simulink model "Final_ShipModel_R19"  (R2019a)
settings: Solver=VariableStepAuto  StartTime=0.0  StopTime=100  RelTol=1e-3
libraries: simulink x3, mssSimulink x2
settings Model: PacingRate=10  Creator=Lenovo  LastModifiedBy=LENOVO
settings DebuggingCC: UnconnectedInputMsg=none  UnconnectedOutputMsg=none  UnconnectedLineMsg=none  SFMachineParentedDataDiag=error

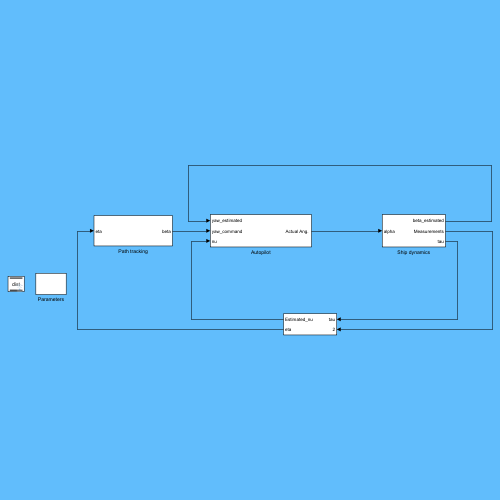
[thumbnail: Simulink's stored preview of the top-level diagram]
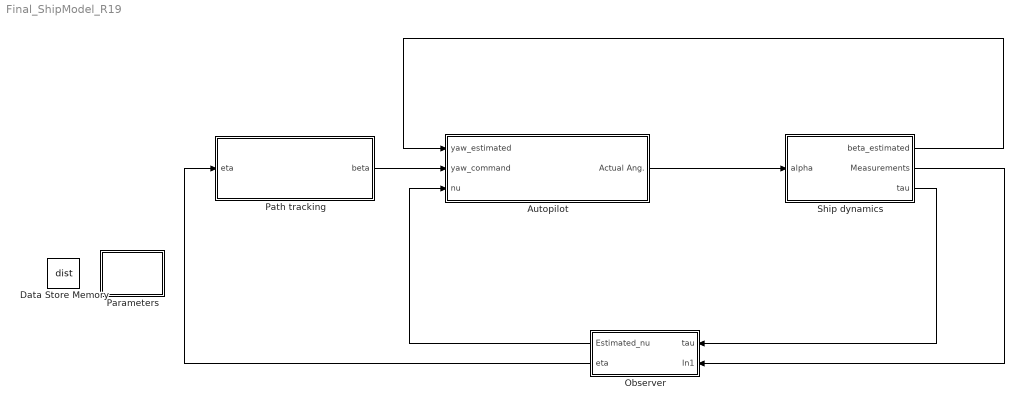
== system Final_ShipModel_R19 ==
  Autopilot : Subsystem
  Data Store Memory : DataStoreMemory  DataStoreName=dist  WriteAfterWriteMsg=warning  InitialValue=1000  ShowAdditionalParam=off  OutDataTypeStr=double
  Observer : Subsystem
  Parameters : Subsystem
  Path tracking : Subsystem
  Ship dynamics : Subsystem
  wires:
  Path tracking/1(beta) -> Autopilot/2(yaw_command)
  Autopilot/1("Actual Ang. ") -> Ship dynamics/1(alpha)
  Ship dynamics/1(beta_estimated) -> Autopilot/1(yaw_estimated)
  Ship dynamics/2(Measurements) -> Observer/2(In1)
  Ship dynamics/3(tau) -> Observer/1(tau)
  Observer/2(eta) -> Path tracking/1(eta)
  Observer/1(Estimated_nu) -> Autopilot/3(nu)

== system Final_ShipModel_R19/Autopilot ==
  yaw_estimated : Inport
  yaw_command : Inport  Port=2
  nu : Inport  Port=3
  Autopilot : Subsystem
  Constant3 : Constant  Value=0
  Fin/Rudder Machinery : Subsystem  AncestorBlock=mssSimulink/Modelling/Control Surfaces/Fin//Rudder Machinery  mask(Rudder Machinery){Dmax=20, Dvmax=2*pi*1000/180, tc=.1}
      mask prompts: Dmax "Max. Rudder Angle (rad):"; Dvmax "Max. Rudder Rate (rad/sec.):"; tc "Time constant (sec):"
      mask help:
      | Model of van Amerongen for rudder machiery
      | Copyright (C) 2005 NTNU
      | Author: Tristan Perez
      mask Help: Rudder machinery model of Van Amerongen accounting for saturation and rate limit.
  Selector : Selector  InputPortWidth=3  IndexOptions=Index vector (dialog)  Indices=[3]  OutputSizes=1
  "Actual Ang. " : Outport
  wires:
  Selector/1 -> Autopilot/4(r_estimated)  "r"
  Constant3/1 -> Autopilot/3(r_command)
  yaw_estimated/1 -> Autopilot/2(yaw_estimated)
  Fin/Rudder Machinery/1("Actual Ang. ") -> "Actual Ang. "/1
  Autopilot/1(rudder_angle_command) -> Fin/Rudder Machinery/1(Angle Comm)
  nu/1 -> Selector/1
  yaw_command/1 -> Autopilot/1(yaw_command)

== system Final_ShipModel_R19/Observer ==
  tau : Inport
  In1 : Inport  Port=2
  Kalman gain : Gain  Gain=-10
  Sensor Model(Supply vessel2) : Subsystem  AncestorBlock=mssSimulink/Marine craft models/Supply vessel
  Sum : Sum  Inputs=-+|
  Estimated_nu : Outport
  eta : Outport  Port=2
  wires:
  Kalman gain/1 -> Sensor Model(Supply vessel2)/2(Error*Kalman Gain)
  Sensor Model(Supply vessel2)/1(Estimated_eta) -> Sum/2, eta/1  "eta"
  In1/1 -> Sum/1
  Sensor Model(Supply vessel2)/2(Estimated_nu) -> Estimated_nu/1
  tau/1 -> Sensor Model(Supply vessel2)/1(tau)
  Sum/1 -> Kalman gain/1

== system Final_ShipModel_R19/Parameters ==
  Izz : Constant  Value=47.934*10^6
  Izz1 : Constant  Value=47.934*10^6*0.8
  Mass : Constant  Value=357.0*1014
  Mass1 : Constant  Value=357.0*1014*0.8
  tag scope: Izz1=global, Izz=global, Mass1=global, Mass=global
  wires:
  Mass/1 -> [Mass]
  Izz/1 -> [Izz]
  Izz1/1 -> [Izz1]
  Mass1/1 -> [Mass1]

== system Final_ShipModel_R19/Path tracking ==
  eta : Inport
  Data Store Read : DataStoreRead  DataStoreName=dist
  Path assigning : MATLAB Function  TreatAsAtomicUnit=on
  Path following : Subsystem
  Path generation : Constant  Value=[500 0; 500 2000; 1000 1500; 2000 0]
  Stop Simulation1 : Stop
  beta : Outport
  wires:
  Path generation/1 -> Path assigning/1(path)
  Data Store Read/1 -> Path assigning/2(dist)
  Path assigning/1(wp1) -> Path following/2(Waypoint 1)
  Path assigning/3(stop) -> Stop Simulation1/1
  Path assigning/2(wp2) -> Path following/3(Waypoint 2)
  eta/1 -> Path following/1(Ship Position)
  Path following/1(beta) -> beta/1

== system Final_ShipModel_R19/Ship dynamics ==
  alpha : Inport
  Noises : Subsystem
  Pod-Propellers : Subsystem
  Supply vessel dynamics : Subsystem
  beta_estimated : Outport
  Measurements : Outport  Port=2
  tau : Outport  Port=3
  wires:
  Pod-Propellers/1(tau) -> Supply vessel dynamics/1(tau), tau/1
  Supply vessel dynamics/3(nu) -> Pod-Propellers/2(nu1)
  Supply vessel dynamics/2(beta_estimated) -> beta_estimated/1
  Noises/1(Noises) -> Measurements/1
  Supply vessel dynamics/1(eta) -> Noises/1(Signal)
  alpha/1 -> Pod-Propellers/1(alpha)

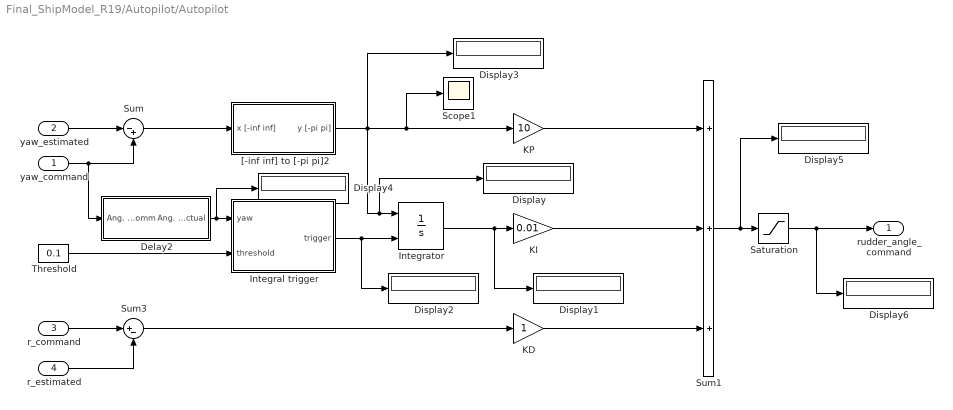
== system Final_ShipModel_R19/Autopilot/Autopilot ==
  yaw_command : Inport
  yaw_estimated : Inport  Port=2
  r_command : Inport  Port=3
  r_estimated : Inport  Port=4
  Delay2 : Subsystem
  Display{,1..6} (7 alike) : Display
  Integral trigger : MATLAB Function  TreatAsAtomicUnit=on
  Integrator : Integrator  ExternalReset=level hold  LimitOutput=on  UpperSaturationLimit=deg2rad(20)  LowerSaturationLimit=deg2rad(-20)
  KD : Gain
  KI : Gain  Gain=0.01
  KP : Gain  Gain=10
  Saturation : Saturate  UpperLimit=deg2rad(20)  LowerLimit=deg2rad(-20)
  Scope1 : Scope
  Sum : Sum  Inputs=|-+
  Sum1 : Sum  Inputs=+++  InputSameDT=on  SaturateOnIntegerOverflow=on  OutDataTypeStr=Inherit: Same as first input
  Sum3 : Sum  Inputs=|+-  InputSameDT=on  SaturateOnIntegerOverflow=on  OutDataTypeStr=Inherit: Same as first input
  Threshold : Constant  Value=0.1
  "[-inf inf] to [-pi pi]2" : Subsystem  AncestorBlock=mssSimulink/Utilities/Math Operations/[-inf inf] to [-pi pi]  mask([-inf inf] to [-pi pi]){}
      mask help: Converts an angle in rad to (-pi pi)
  rudder_angle_command : Outport
  wires:
  Integrator/1 -> Display1/1, KI/1
  KD/1 -> Sum1/3
  Sum/1 -> "[-inf inf] to [-pi pi]2"/1(x [-inf inf])
  Sum3/1 -> KD/1
  "[-inf inf] to [-pi pi]2"/1(y [-pi pi]) -> Scope1/1, KP/1, Display3/1, Display/1, Integrator/1
  KI/1 -> Sum1/2
  Sum1/1 -> Display5/1, Saturation/1
  r_estimated/1 -> Sum3/2
  r_command/1 -> Sum3/1
  yaw_estimated/1 -> Sum/1
  KP/1 -> Sum1/1
  Integral trigger/1(trigger) -> Display2/1, Integrator/2
  Threshold/1 -> Integral trigger/2(threshold)
  yaw_command/1 -> Sum/2, Delay2/1(Ang. Comm)
  Delay2/1(Ang. Actual) -> Display4/1, Integral trigger/1(yaw)
  Saturation/1 -> Display6/1, rudder_angle_command/1

== system Final_ShipModel_R19/Autopilot/Fin//Rudder Machinery ==
  Angle Comm : Inport
  Gain : Gain  Gain=1/tc  SaturateOnIntegerOverflow=on  OutDataTypeStr=Inherit: Same as input  ParamDataTypeStr=Inherit: Same as input
  Gain1 : Gain  Gain=-1
  Integrator : Integrator
  Saturation : Saturate  UpperLimit=deg2rad(30)  LowerLimit=-deg2rad(30)
  Saturation1 : Saturate  UpperLimit=deg2rad(Dmax)  LowerLimit=deg2rad(-Dmax)
  Sum : Sum  Inputs=|+-  InputSameDT=on  SaturateOnIntegerOverflow=on  OutDataTypeStr=Inherit: Same as first input
  "Actual Ang. " : Outport  VectorParamsAs1DForOutWhenUnconnected=off
  wires:
  Gain/1 -> Saturation/1
  Sum/1 -> Gain/1
  Integrator/1 -> Sum/2, Gain1/1
  Saturation1/1 -> Sum/1
  Saturation/1 -> Integrator/1
  Angle Comm/1 -> Saturation1/1
  Gain1/1 -> "Actual Ang. "/1

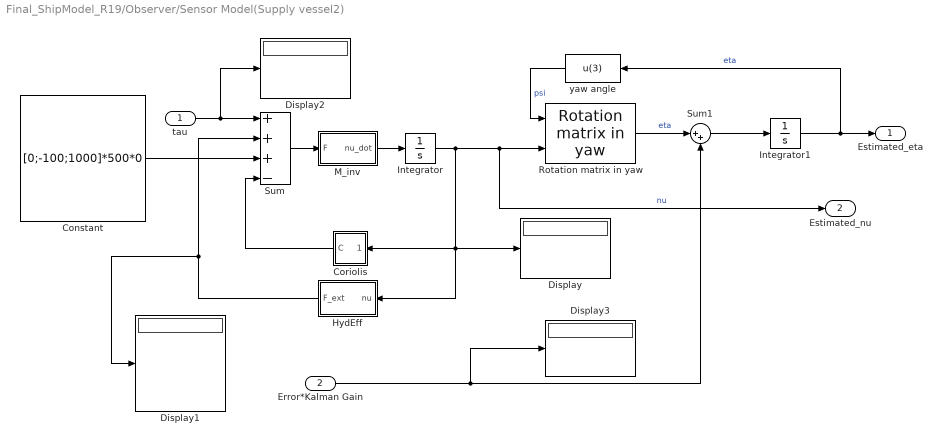
== system Final_ShipModel_R19/Observer/Sensor Model(Supply vessel2) ==
  tau : Inport
  Error*Kalman Gain : Inport  Port=2
  Constant : Constant  Value=[0;-100;1000]*500*0
  Coriolis : Subsystem
  Display{,1..3} (4 alike) : Display
  HydEff : Subsystem
  Integrator : Integrator  InitialCondition=[0 1 0]
  Integrator1 : Integrator
  M_inv : Subsystem
  "Rotation matrix in yaw " : mssSimulink/Modelling/Kinematics/Rotation matrix in yaw 
  Sum : Sum  Inputs=+++-  InputSameDT=on  SaturateOnIntegerOverflow=on  OutDataTypeStr=Inherit: Same as first input
  Sum1 : Sum  Inputs=|++
  yaw angle : Fcn  Expr=u(3)
  Estimated_eta : Outport  InitialOutput=0  VectorParamsAs1DForOutWhenUnconnected=off
  Estimated_nu : Outport  Port=2  InitialOutput=0  VectorParamsAs1DForOutWhenUnconnected=off
  wires:
  Sum/1 -> M_inv/1(F)
  M_inv/1(nu_dot) -> Integrator/1
  tau/1 -> Display2/1, Sum/1
  yaw angle/1 -> "Rotation matrix in yaw "/1  "psi"
  Integrator/1 -> Estimated_nu/1, "Rotation matrix in yaw "/2, Display/1, HydEff/1(nu), Coriolis/1(nu)  "nu"
  HydEff/1(F_ext) -> Display1/1, Sum/2
  Coriolis/1(C) -> Sum/4
  Constant/1 -> Sum/3
  Integrator1/1 -> Estimated_eta/1, yaw angle/1  "eta"
  Error*Kalman Gain/1 -> Display3/1, Sum1/2
  Sum1/1 -> Integrator1/1
  "Rotation matrix in yaw "/1 -> Sum1/1  "eta"

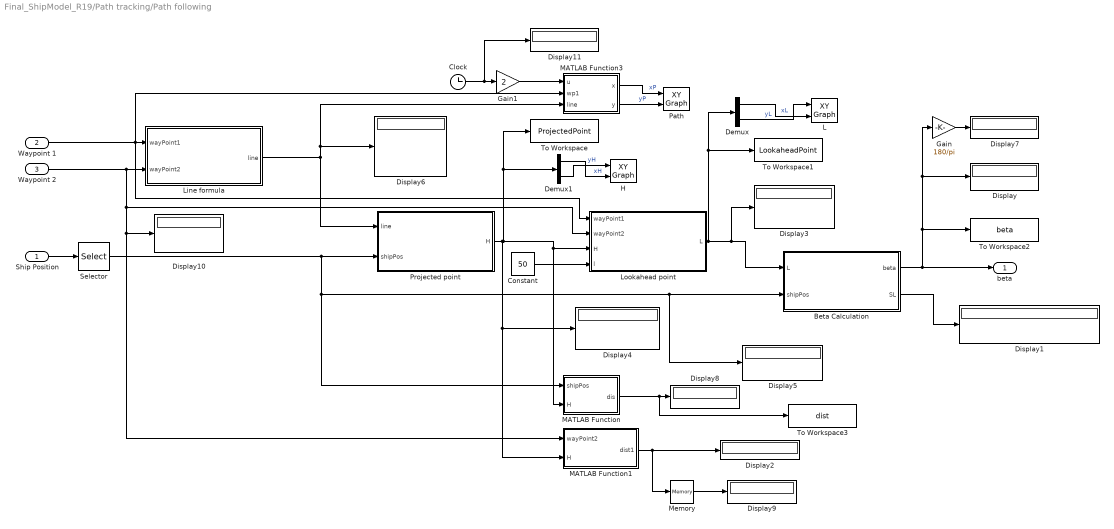
== system Final_ShipModel_R19/Path tracking/Path following ==
  Ship Position : Inport
  Waypoint 1 : Inport  Port=2
  Waypoint 2 : Inport  Port=3
  Beta Calculation : MATLAB Function  TreatAsAtomicUnit=on
  Clock : Clock
  Constant : Constant  Value=50
  Demux : Demux  Outputs=2
  Demux1 : Demux  Outputs=2
  Display{,1..11} (12 alike) : Display
  Gain : Gain  Gain=180/pi
  Gain1 : Gain  Gain=2
  H : simulink/Sinks/XY Graph  xmin=-1  xmax=1  ymin=-1  ymax=1  st=-1
  L : simulink/Sinks/XY Graph  xmin=-1  xmax=1  ymin=-1  ymax=1  st=-1
  Line formula : MATLAB Function  TreatAsAtomicUnit=on
  Lookahead point : MATLAB Function  TreatAsAtomicUnit=on
  MATLAB Function : MATLAB Function  TreatAsAtomicUnit=on
  MATLAB Function1 : MATLAB Function  TreatAsAtomicUnit=on
  MATLAB Function3 : MATLAB Function  TreatAsAtomicUnit=on
  Memory : Memory
  Path : simulink/Sinks/XY Graph  xmin=-1  xmax=1  ymin=-1  ymax=1  st=-1
  Projected point : MATLAB Function  TreatAsAtomicUnit=on
  Selector : Selector  InputPortWidth=3  IndexOptions=Index vector (dialog)  Indices=[1 2]  OutputSizes=1
  To Workspace : ToWorkspace  VariableName=ProjectedPoint  SaveFormat=Timeseries  SampleTime=-1
  To Workspace1 : ToWorkspace  VariableName=LookaheadPoint  SaveFormat=Timeseries  SampleTime=-1
  To Workspace2 : ToWorkspace  VariableName=beta  SaveFormat=Timeseries  SampleTime=-1
  To Workspace3 : ToWorkspace  VariableName=dist  SaveFormat=Timeseries  SampleTime=-1
  beta : Outport
  wires:
  Waypoint 1/1 -> Lookahead point/1(wayPoint1), Line formula/1(wayPoint1), MATLAB Function3/2(wp1)
  Waypoint 2/1 -> MATLAB Function1/1(wayPoint2), Display10/1, Lookahead point/2(wayPoint2), Line formula/2(wayPoint2)
  Ship Position/1 -> Selector/1
  Projected point/1(H) -> Display4/1, MATLAB Function1/2(H), To Workspace/1, Demux1/1, MATLAB Function/2(H), Lookahead point/3(H)
  Constant/1 -> Lookahead point/4(l)
  Lookahead point/1(L) -> To Workspace1/1, Demux/1, Display3/1, Beta Calculation/1(L)
  Beta Calculation/1(beta) -> beta/1, To Workspace2/1, Display/1, Gain/1
  Beta Calculation/2(SL) -> Display1/1
  Selector/1 -> Display5/1, Beta Calculation/2(shipPos), MATLAB Function/1(shipPos), Projected point/2(shipPos)
  Gain/1 -> Display7/1
  Gain1/1 -> MATLAB Function3/1(u)
  Clock/1 -> Display11/1, Gain1/1
  Line formula/1(line) -> Projected point/1(line), MATLAB Function3/3(line), Display6/1
  MATLAB Function3/2(y) -> Path/2  "yP"
  Demux/1 -> L/2  "xL"
  Demux/2 -> L/1  "yL"
  Demux1/1 -> H/2  "xH"
  Demux1/2 -> H/1  "yH"
  MATLAB Function/1(dis) -> To Workspace3/1, Display8/1
  MATLAB Function3/1(x) -> Path/1  "xP"
  MATLAB Function1/1(dist1) -> Display2/1, Memory/1
  Memory/1 -> Display9/1

== system Final_ShipModel_R19/Ship dynamics/Noises ==
  Signal : Inport
  Amplitude : Constant  Value=0
  Clock : Clock
  Mux1 : Mux  Inputs=3
  Sine Wave : Sin  TimeSource=Use external signal  Frequency=2  SampleTime=0
  Sum1 : Sum  Inputs=|++
  Noises : Outport
  wires:
  Signal/1 -> Sum1/1
  Clock/1 -> Sine Wave/1
  Sine Wave/1 -> Mux1/1, Mux1/2
  Sum1/1 -> Noises/1
  Mux1/1 -> Sum1/2
  Amplitude/1 -> Mux1/3

== system Final_ShipModel_R19/Ship dynamics/Pod-Propellers ==
  alpha : Inport
  nu1 : Inport  Port=2
  Add : Sum
  Propeller speed : Constant  Value=200
  propL : Subsystem
  propR : Subsystem
  tau : Outport
  wires:
  nu1/1 -> propL/1(nu), propR/1(nu1)
  alpha/1 -> propR/2(alpha1), propL/2(alpha)
  Propeller speed/1 -> propL/3(RPM), propR/3(RPM1)
  Add/1 -> tau/1
  propL/1(tau) -> Add/2
  propR/1(tau1) -> Add/1

== system Final_ShipModel_R19/Ship dynamics/Supply vessel dynamics ==
  tau : Inport
  MATLAB Function : MATLAB Function  TreatAsAtomicUnit=on
  Supply vessel : Subsystem  AncestorBlock=mssSimulink/Marine craft models/Supply vessel
  eta : Outport
  beta_estimated : Outport  Port=2
  nu : Outport  Port=3
  wires:
  MATLAB Function/1(beta_estimated) -> beta_estimated/1
  Supply vessel/3(velo) -> MATLAB Function/1(velo)
  tau/1 -> Supply vessel/1(tau)
  Supply vessel/1(eta) -> eta/1  "eta"
  Supply vessel/2(nu) -> nu/1

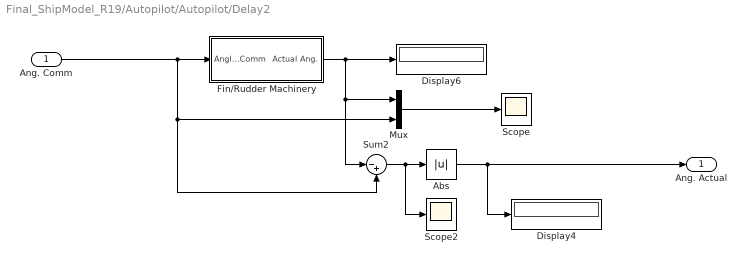
== system Final_ShipModel_R19/Autopilot/Autopilot/Delay2 ==
  Ang. Comm : Inport
  Abs : Abs  ZeroCross=off
  Display4 : Display
  Display6 : Display
  Fin/Rudder Machinery : Subsystem  AncestorBlock=mssSimulink/Modelling/Control Surfaces/Fin//Rudder Machinery  mask(Rudder Machinery){Dmax=20, Dvmax=0.05, tc=.005}
      mask prompts: Dmax "Max. Rudder Angle (rad):"; Dvmax "Max. Rudder Rate (rad/sec.):"; tc "Time constant (sec):"
      mask help:
      | Model of van Amerongen for rudder machiery
      | Copyright (C) 2005 NTNU
      | Author: Tristan Perez
      mask Help: Rudder machinery model of Van Amerongen accounting for saturation and rate limit.
  Mux : Mux  Inputs=2
  Scope : Scope
  Scope2 : Scope
  Sum2 : Sum  Inputs=|-+
  Ang. Actual : Outport
  wires:
  Sum2/1 -> Scope2/1, Abs/1
  Ang. Comm/1 -> Fin/Rudder Machinery/1(Angle Comm), Sum2/2, Mux/2
  Fin/Rudder Machinery/1("Actual Ang. ") -> Sum2/1, Mux/1, Display6/1
  Abs/1 -> Ang. Actual/1, Display4/1
  Mux/1 -> Scope/1

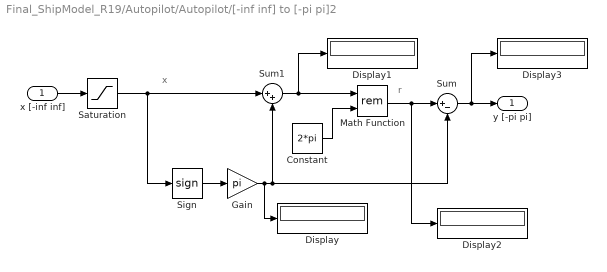
== system Final_ShipModel_R19/Autopilot/Autopilot/[-inf inf] to [-pi pi]2 ==
  note: x
  note: r
  x [-inf inf] : Inport
  Constant : Constant  Value=2*pi
  Display{,1..3} (4 alike) : Display
  Gain : Gain  Gain=pi  SaturateOnIntegerOverflow=on  OutDataTypeStr=Inherit: Same as input  ParamDataTypeStr=Inherit: Same as input
  Math Function : Math  Operator=rem  SaturateOnIntegerOverflow=on
  Saturation : Saturate  UpperLimit=1e10  LowerLimit=-1e10
  Sign : Signum
  Sum : Sum  Inputs=|+-  SaturateOnIntegerOverflow=on
  Sum1 : Sum  Inputs=|++  SaturateOnIntegerOverflow=on
  y [-pi pi] : Outport  VectorParamsAs1DForOutWhenUnconnected=off
  wires:
  x [-inf inf]/1 -> Saturation/1
  Sign/1 -> Gain/1
  Gain/1 -> Display/1, Sum/2, Sum1/2
  Sum1/1 -> Display1/1, Math Function/1
  Constant/1 -> Math Function/2
  Sum/1 -> Display3/1, y [-pi pi]/1
  Saturation/1 -> Sum1/1, Sign/1
  Math Function/1 -> Display2/1, Sum/1

== system Final_ShipModel_R19/Observer/Sensor Model(Supply vessel2)/Coriolis ==
  nu : Inport
  Demux : Demux  Outputs=3
  Display : Display
  MATLAB Function : MATLAB Function  TreatAsAtomicUnit=on
  Mux : Mux  Inputs=3
  C : Outport
  wires:
  nu/1 -> Display/1, Demux/1
  MATLAB Function/2(C2) -> Mux/2
  MATLAB Function/3(C3) -> Mux/3
  MATLAB Function/1(C1) -> Mux/1
  Mux/1 -> C/1
  Demux/1 -> MATLAB Function/1(u)
  Demux/2 -> MATLAB Function/2(v)
  Demux/3 -> MATLAB Function/3(r)

== system Final_ShipModel_R19/Observer/Sensor Model(Supply vessel2)/HydEff ==
  nu : Inport
  Bus Creator : BusCreator  Inputs=3
  Demux : Demux  Outputs=3
  MATLAB Function : MATLAB Function  TreatAsAtomicUnit=on
  F_ext : Outport
  wires:
  [Mass1] -> MATLAB Function/1(mass)
  MATLAB Function/1(Xh) -> Bus Creator/1
  Bus Creator/1 -> F_ext/1
  MATLAB Function/2(Yh) -> Bus Creator/2
  MATLAB Function/3(Nh) -> Bus Creator/3
  nu/1 -> Demux/1
  Demux/1 -> MATLAB Function/2(u)
  Demux/2 -> MATLAB Function/3(v)
  Demux/3 -> MATLAB Function/4(r)

== system Final_ShipModel_R19/Observer/Sensor Model(Supply vessel2)/M_inv ==
  F : Inport
  Display : Display
  MATLAB Function : MATLAB Function  TreatAsAtomicUnit=on
  Matrix Multiply : Product  Multiplication=Matrix(*)
  nu_dot : Outport
  wires:
  MATLAB Function/1(Minv) -> Display/1, Matrix Multiply/2
  [Mass] -> MATLAB Function/1(mass)
  [Izz] -> MATLAB Function/2(Izz)
  Matrix Multiply/1 -> nu_dot/1
  F/1 -> Matrix Multiply/1

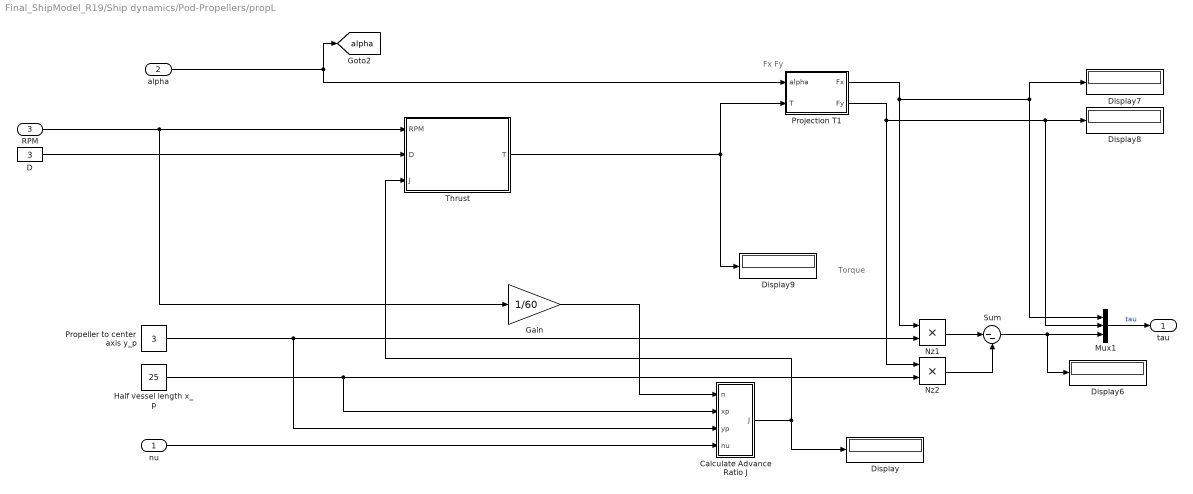
== system Final_ShipModel_R19/Ship dynamics/Pod-Propellers/propL ==
  note: Fx Fy
  note: Torque
  nu : Inport
  alpha : Inport  Port=2
  RPM : Inport  Port=3
  Calculate Advance Ratio J : Subsystem
  D : Constant  Value=3
  Display{,6..9} (5 alike) : Display
  Gain : Gain  Gain=1/60
  Half vessel length x_p : Constant  Value=25
  Mux1 : Mux  Inputs=3
  Nz1 : Product
  Nz2 : Product
  Projection T1 : MATLAB Function  TreatAsAtomicUnit=on
  Propeller to center axis y_p : Constant  Value=3
  Sum : Sum  Inputs=|--
  Thrust : Subsystem
  tau : Outport
  tag scope: alpha=global
  wires:
  Gain/1 -> Calculate Advance Ratio J/1(n)
  Thrust/1(T) -> Projection T1/2(T), Display9/1
  Propeller to center axis y_p/1 -> Calculate Advance Ratio J/3(yp), Nz1/2
  Projection T1/2(Fy) -> Mux1/2, Display8/1, Nz2/1
  RPM/1 -> Gain/1, Thrust/1(RPM)
  Nz2/1 -> Sum/2
  Projection T1/1(Fx) -> Display7/1, Mux1/1, Nz1/1
  Mux1/1 -> tau/1  "tau"
  alpha/1 -> Projection T1/1(alpha), [alpha]
  D/1 -> Thrust/2(D)
  nu/1 -> Calculate Advance Ratio J/4(nu)
  Half vessel length x_p/1 -> Calculate Advance Ratio J/2(xp), Nz2/2
  Nz1/1 -> Sum/1
  Calculate Advance Ratio J/1(J) -> Thrust/3(J), Display/1
  Sum/1 -> Display6/1, Mux1/3

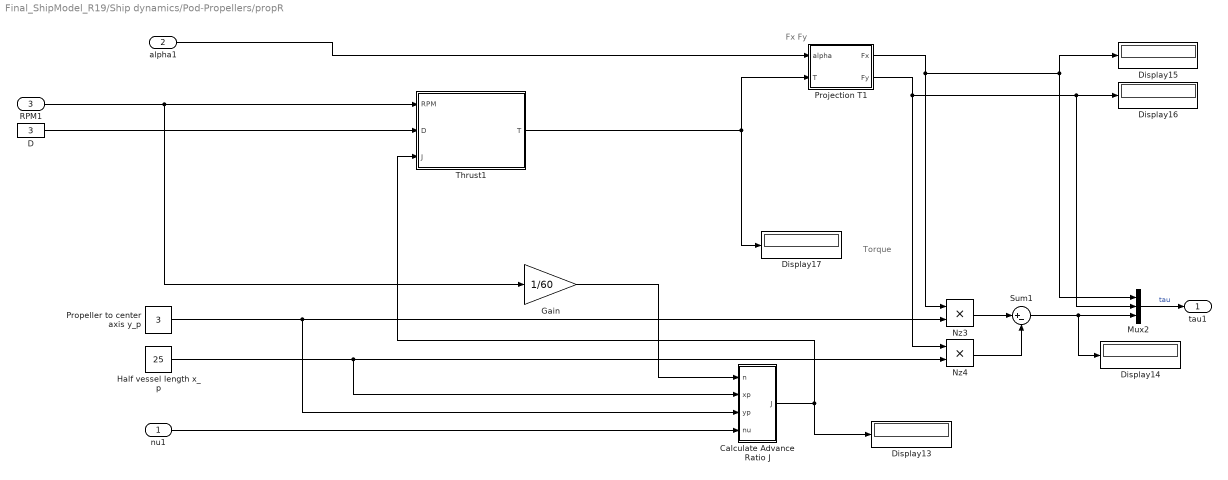
== system Final_ShipModel_R19/Ship dynamics/Pod-Propellers/propR ==
  note: Fx Fy
  note: Torque
  nu1 : Inport
  alpha1 : Inport  Port=2
  RPM1 : Inport  Port=3
  Calculate Advance Ratio J : Subsystem
  D : Constant  Value=3
  Display{13..17} (5 alike) : Display
  Gain : Gain  Gain=1/60
  Half vessel length x_p : Constant  Value=25
  Mux2 : Mux  Inputs=3
  Nz3 : Product
  Nz4 : Product
  Projection T1 : MATLAB Function  TreatAsAtomicUnit=on
  Propeller to center axis y_p : Constant  Value=3
  Sum1 : Sum  Inputs=|+-
  Thrust1 : Subsystem
  tau1 : Outport
  wires:
  Gain/1 -> Calculate Advance Ratio J/1(n)
  Thrust1/1(T) -> Projection T1/2(T), Display17/1
  Propeller to center axis y_p/1 -> Calculate Advance Ratio J/3(yp), Nz3/2
  Projection T1/2(Fy) -> Mux2/2, Display16/1, Nz4/1
  RPM1/1 -> Gain/1, Thrust1/1(RPM)
  Nz4/1 -> Sum1/2
  Projection T1/1(Fx) -> Display15/1, Mux2/1, Nz3/1
  Mux2/1 -> tau1/1  "tau"
  alpha1/1 -> Projection T1/1(alpha)
  D/1 -> Thrust1/2(D)
  nu1/1 -> Calculate Advance Ratio J/4(nu)
  Half vessel length x_p/1 -> Calculate Advance Ratio J/2(xp), Nz4/2
  Nz3/1 -> Sum1/1
  Calculate Advance Ratio J/1(J) -> Thrust1/3(J), Display13/1
  Sum1/1 -> Display14/1, Mux2/3

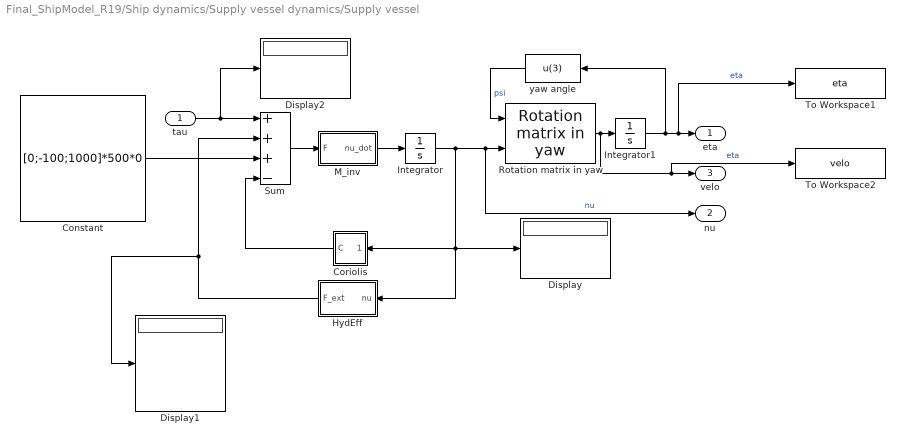
== system Final_ShipModel_R19/Ship dynamics/Supply vessel dynamics/Supply vessel ==
  tau : Inport
  Constant : Constant  Value=[0;-100;1000]*500*0
  Coriolis : Subsystem
  Display : Display
  Display1 : Display
  Display2 : Display
  HydEff : Subsystem
  Integrator : Integrator  InitialCondition=[0 1 0]
  Integrator1 : Integrator
  M_inv : Subsystem
  "Rotation matrix in yaw " : mssSimulink/Modelling/Kinematics/Rotation matrix in yaw 
  Sum : Sum  Inputs=+++-  InputSameDT=on  SaturateOnIntegerOverflow=on  OutDataTypeStr=Inherit: Same as first input
  To Workspace1 : ToWorkspace  VariableName=eta  SaveFormat=Timeseries  SampleTime=-1
  To Workspace2 : ToWorkspace  VariableName=velo  SaveFormat=Timeseries  SampleTime=-1
  yaw angle : Fcn  Expr=u(3)
  eta : Outport  InitialOutput=0  VectorParamsAs1DForOutWhenUnconnected=off
  nu : Outport  Port=2  InitialOutput=0  VectorParamsAs1DForOutWhenUnconnected=off
  velo : Outport  Port=3
  wires:
  Sum/1 -> M_inv/1(F)
  M_inv/1(nu_dot) -> Integrator/1
  tau/1 -> Display2/1, Sum/1
  yaw angle/1 -> "Rotation matrix in yaw "/1  "psi"
  Integrator/1 -> Display/1, HydEff/1(nu), Coriolis/1(nu), "Rotation matrix in yaw "/2, nu/1  "nu"
  HydEff/1(F_ext) -> Display1/1, Sum/2
  Coriolis/1(C) -> Sum/4
  Constant/1 -> Sum/3
  Integrator1/1 -> yaw angle/1, To Workspace1/1, eta/1  "eta"
  "Rotation matrix in yaw "/1 -> To Workspace2/1, velo/1, Integrator1/1  "eta"

== system Final_ShipModel_R19/Autopilot/Autopilot/Delay2/Fin//Rudder Machinery ==
  Angle Comm : Inport
  Gain : Gain  Gain=1/tc  SaturateOnIntegerOverflow=on  OutDataTypeStr=Inherit: Same as input  ParamDataTypeStr=Inherit: Same as input
  Integrator : Integrator
  Saturation : Saturate  UpperLimit=Dvmax  LowerLimit=-Dvmax
  Saturation1 : Saturate  UpperLimit=Dmax  LowerLimit=-Dmax
  Sum : Sum  Inputs=|+-  InputSameDT=on  SaturateOnIntegerOverflow=on  OutDataTypeStr=Inherit: Same as first input
  "[-inf inf] to [-pi pi]" : Subsystem  AncestorBlock=mssSimulink/Utilities/Math Operations/[-inf inf] to [-pi pi]  mask([-inf inf] to [-pi pi]){}
      mask help: Converts an angle in rad to (-pi pi)
  "Actual Ang. " : Outport  VectorParamsAs1DForOutWhenUnconnected=off
  wires:
  Gain/1 -> Saturation/1
  Sum/1 -> Gain/1
  Integrator/1 -> Sum/2, "Actual Ang. "/1
  Saturation1/1 -> Sum/1
  Saturation/1 -> Integrator/1
  Angle Comm/1 -> "[-inf inf] to [-pi pi]"/1(x [-inf inf])
  "[-inf inf] to [-pi pi]"/1(y [-pi pi]) -> Saturation1/1

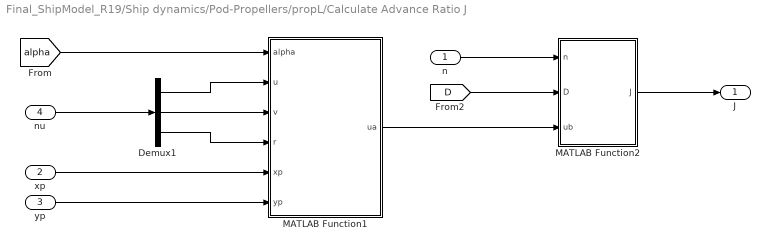
== system Final_ShipModel_R19/Ship dynamics/Pod-Propellers/propL/Calculate Advance Ratio J ==
  n : Inport
  xp : Inport  Port=2
  yp : Inport  Port=3
  nu : Inport  Port=4
  Demux1 : Demux  Outputs=3
  MATLAB Function1 : MATLAB Function  TreatAsAtomicUnit=on
  MATLAB Function2 : MATLAB Function  TreatAsAtomicUnit=on
  J : Outport
  wires:
  Demux1/3 -> MATLAB Function1/4(r)
  Demux1/2 -> MATLAB Function1/3(v)
  n/1 -> MATLAB Function2/1(n)
  nu/1 -> Demux1/1
  MATLAB Function1/1(ua) -> MATLAB Function2/3(ub)
  Demux1/1 -> MATLAB Function1/2(u)
  [D] -> MATLAB Function2/2(D)
  MATLAB Function2/1(J) -> J/1
  xp/1 -> MATLAB Function1/5(xp)
  yp/1 -> MATLAB Function1/6(yp)
  [alpha] -> MATLAB Function1/1(alpha)

== system Final_ShipModel_R19/Ship dynamics/Pod-Propellers/propL/Thrust ==
  RPM : Inport
  D : Inport  Port=2
  J : Inport  Port=3
  1-D Lookup Table : Lookup_n-D  NumberOfTableDimensions=1  BreakpointsForDimension1=[0:0.05:1.05]  Table=-0.3*[0:0.05:1.05]+0.35  InternalRulePriority=Speed  RndMeth=Simplest  InputSameDT=on
  Display12 : Display
  MATLAB Function : MATLAB Function  TreatAsAtomicUnit=on
  T : Outport
  wires:
  1-D Lookup Table/1 -> MATLAB Function/3(K_T), Display12/1
  D/1 -> MATLAB Function/2(D)
  MATLAB Function/1(T) -> T/1
  J/1 -> 1-D Lookup Table/1
  RPM/1 -> MATLAB Function/1(RPM)

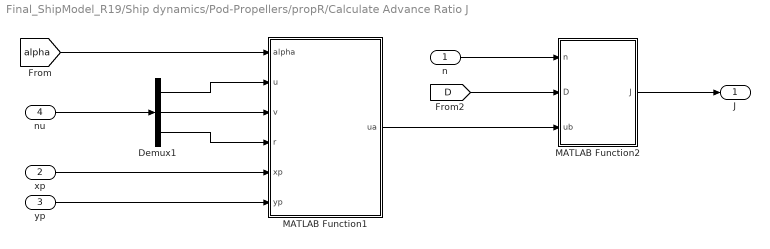
== system Final_ShipModel_R19/Ship dynamics/Pod-Propellers/propR/Calculate Advance Ratio J ==
  n : Inport
  xp : Inport  Port=2
  yp : Inport  Port=3
  nu : Inport  Port=4
  Demux1 : Demux  Outputs=3
  MATLAB Function1 : MATLAB Function  TreatAsAtomicUnit=on
  MATLAB Function2 : MATLAB Function  TreatAsAtomicUnit=on
  J : Outport
  wires:
  Demux1/3 -> MATLAB Function1/4(r)
  Demux1/2 -> MATLAB Function1/3(v)
  n/1 -> MATLAB Function2/1(n)
  nu/1 -> Demux1/1
  MATLAB Function1/1(ua) -> MATLAB Function2/3(ub)
  Demux1/1 -> MATLAB Function1/2(u)
  [D] -> MATLAB Function2/2(D)
  MATLAB Function2/1(J) -> J/1
  xp/1 -> MATLAB Function1/5(xp)
  yp/1 -> MATLAB Function1/6(yp)
  [alpha] -> MATLAB Function1/1(alpha)

== system Final_ShipModel_R19/Ship dynamics/Pod-Propellers/propR/Thrust1 ==
  RPM : Inport
  D : Inport  Port=2
  J : Inport  Port=3
  1-D Lookup Table : Lookup_n-D  NumberOfTableDimensions=1  BreakpointsForDimension1=[0:0.05:1.05]  Table=-0.3*[0:0.05:1.05]+0.35  InternalRulePriority=Speed  RndMeth=Simplest  InputSameDT=on
  Display12 : Display
  MATLAB Function : MATLAB Function  TreatAsAtomicUnit=on
  T : Outport
  tag scope: D=global
  wires:
  1-D Lookup Table/1 -> MATLAB Function/3(K_T), Display12/1
  D/1 -> [D], MATLAB Function/2(D)
  MATLAB Function/1(T) -> T/1
  J/1 -> 1-D Lookup Table/1
  RPM/1 -> MATLAB Function/1(RPM)

== system Final_ShipModel_R19/Ship dynamics/Supply vessel dynamics/Supply vessel/Coriolis ==
  nu : Inport
  Demux : Demux  Outputs=3
  Display : Display
  MATLAB Function : MATLAB Function  TreatAsAtomicUnit=on
  Mux : Mux  Inputs=3
  C : Outport
  wires:
  nu/1 -> Display/1, Demux/1
  MATLAB Function/2(C2) -> Mux/2
  MATLAB Function/3(C3) -> Mux/3
  MATLAB Function/1(C1) -> Mux/1
  Mux/1 -> C/1
  Demux/1 -> MATLAB Function/1(u)
  Demux/2 -> MATLAB Function/2(v)
  Demux/3 -> MATLAB Function/3(r)

== system Final_ShipModel_R19/Ship dynamics/Supply vessel dynamics/Supply vessel/HydEff ==
  nu : Inport
  Bus Creator : BusCreator  Inputs=3
  Demux : Demux  Outputs=3
  MATLAB Function : MATLAB Function  TreatAsAtomicUnit=on
  F_ext : Outport
  wires:
  [Mass] -> MATLAB Function/1(mass)
  MATLAB Function/1(Xh) -> Bus Creator/1
  Bus Creator/1 -> F_ext/1
  MATLAB Function/2(Yh) -> Bus Creator/2
  MATLAB Function/3(Nh) -> Bus Creator/3
  nu/1 -> Demux/1
  Demux/1 -> MATLAB Function/2(u)
  Demux/2 -> MATLAB Function/3(v)
  Demux/3 -> MATLAB Function/4(r)

== system Final_ShipModel_R19/Ship dynamics/Supply vessel dynamics/Supply vessel/M_inv ==
  F : Inport
  Display : Display
  MATLAB Function : MATLAB Function  TreatAsAtomicUnit=on
  Matrix Multiply : Product  Multiplication=Matrix(*)
  nu_dot : Outport
  wires:
  MATLAB Function/1(Minv) -> Display/1, Matrix Multiply/2
  [Mass] -> MATLAB Function/1(mass)
  [Izz] -> MATLAB Function/2(Izz)
  Matrix Multiply/1 -> nu_dot/1
  F/1 -> Matrix Multiply/1

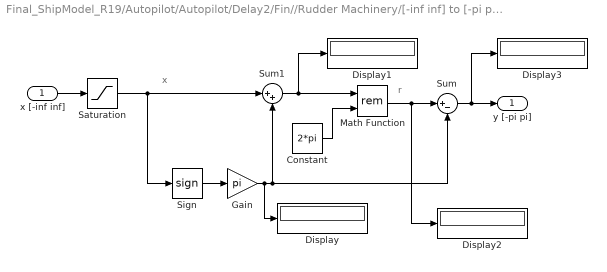
== system Final_ShipModel_R19/Autopilot/Autopilot/Delay2/Fin//Rudder Machinery/[-inf inf] to [-pi pi] ==
  note: x
  note: r
  x [-inf inf] : Inport
  Constant : Constant  Value=2*pi
  Display{,1..3} (4 alike) : Display
  Gain : Gain  Gain=pi  SaturateOnIntegerOverflow=on  OutDataTypeStr=Inherit: Same as input  ParamDataTypeStr=Inherit: Same as input
  Math Function : Math  Operator=rem  SaturateOnIntegerOverflow=on
  Saturation : Saturate  UpperLimit=1e10  LowerLimit=-1e10
  Sign : Signum
  Sum : Sum  Inputs=|+-  SaturateOnIntegerOverflow=on
  Sum1 : Sum  Inputs=|++  SaturateOnIntegerOverflow=on
  y [-pi pi] : Outport  VectorParamsAs1DForOutWhenUnconnected=off
  wires:
  x [-inf inf]/1 -> Saturation/1
  Sign/1 -> Gain/1
  Gain/1 -> Display/1, Sum/2, Sum1/2
  Sum1/1 -> Display1/1, Math Function/1
  Constant/1 -> Math Function/2
  Sum/1 -> Display3/1, y [-pi pi]/1
  Saturation/1 -> Sum1/1, Sign/1
  Math Function/1 -> Display2/1, Sum/1

== matlab function Final_ShipModel_R19/Ship dynamics/Supply vessel dynamics/Supply vessel/Coriolis/MATLAB Function ==
  data: u input; C1 output; C2 output; C3 output; v input; r input
function [C1,    C2,    C3]    = fcn(u,v,r)

% u = nu(1);
% v = nu(2);
% r = nu(3);

x_g = 0;
m = 357.0*1014;

C = [0                 0  -m*(x_g*r + v); ...
     0                 0             m*u; ...
     m*(x_g*r + v)  -m*u              0];

Co = C*[u;v;r];
C1 = Co(1);
C2 = Co(2);
C3 = Co(3);

end

% Xc =   h.m*(r*v+h.xG*r^2-h.zG*p*r);  
% Yc = - h.m*u*r;
% Kc =   h.m*h.zG*u*r;
% Nc = - h.m*h.xG*u*r;

== matlab function Final_ShipModel_R19/Ship dynamics/Pod-Propellers/propL/Calculate Advance Ratio J/MATLAB Function1 ==
  data: alpha input; u input; v input; ua output; r input; xp input; yp input
function ua = fcn(alpha, u, v ,r , xp , yp)
    
    uax = u + yp*r;     % Uax is velocity of propeller projected on x
    uay = v - xp*r;     % Uay is velocity of propeller projected on y
    phi = atan(uay/uax);    % Angle between ship velocity and x axis
    beta = phi - alpha;     % Angle difference between ship velocity and propeller's thrust

    ua = abs(hypot(uax,uay)*cos(beta)); % project ua on direction velocity of ship
end

== matlab function Final_ShipModel_R19/Ship dynamics/Supply vessel dynamics/Supply vessel/M_inv/MATLAB Function ==
  data: Minv output; mass input; Izz input
function Minv = fcn(mass, Izz)

h.m   = mass;    % Mass [Kg]
h.Izz = Izz;     % Yaw Inertia
h.xG  = 0;

%%%%%%%%%%%%%%%%%%%%%%%%%%%%%%%%%%%%%%%%%%%%%%%%%%%%%%%%%%%%%%%%%%%%%%%
% The hydrodynamic derivatives are given in dimensional form, and follow
% from the original publication of Blanke and Christensen 1993.
%%%%%%%%%%%%%%%%%%%%%%%%%%%%%%%%%%%%%%%%%%%%%%%%%%%%%%%%%%%%%%%%%%%%%%%
% Data for surge equation 
h.Xudot  	= -17400.0;
% h.Xuau     	= -1.96e+003;
% h.Xvr    	=  0.33 * mass;
   
% Hydrodynamic coefficients in sway equation
h.Yvdot = -393000; 
h.Ypdot = -296000; 
h.Yrdot = -1400000; 
% h.Yauv  = -11800; 
% h.Yur   =  131000; 
% h.Yvav  = -3700; 
% h.Yrar  =  0;
% h.Yvar  = -794000; 
% h.Yrav  = -182000; 
% h.Ybauv =  10800; % Y_{\phi |v u|}
% h.Ybaur =  251000; 
% h.Ybuu  = -74;


% Hydrodynamic coefficients in yaw equation
h.Nvdot =  538000;
h.Npdot =  0;
h.Nrdot = -38.7e6;
% h.Nauv  = -92000;
% h.Naur  = -4710000;
% h.Nvav  =  0;
% h.Nrar  = -202000000;
% h.Nvar  =  0;
% h.Nrav  = -15600000;
% h.Nbauv = -214000;
% h.Nbuar = -4980000;
% h.Nbuau = -8000;
%%%%%%%%%%%%%%%%%%%%%%%%%%%%%%%%%%%%%%%%%%%%%%%%%%%%%%%%%%%%%%%%%%%%%%%%%%%


M = [(h.m-h.Xudot)                  0                  0; ...
                 0      (h.m-h.Yvdot) (h.m*h.xG-h.Yrdot); ...
                 0 (h.m*h.xG-h.Nvdot)    (h.Izz-h.Nrdot)];

Minv = inv(M);
end

== matlab function Final_ShipModel_R19/Ship dynamics/Supply vessel dynamics/Supply vessel/HydEff/MATLAB Function ==
  data: mass input; Xh output; Yh output; Nh output; u input; v input; r input
function [Xh, Yh, Nh] = fcn(mass, u, v, r)

%%%%%%%%%%%%%%%%%%%%%%%%%%%%%%%%%%%%%%%%%%%%%%%%%%%%%%%%%%%%%%%%%%%%%%%
% The hydrodynamic derivatives are given in dimensional form, and follow
% from the original publication of Blanke and Christensen 1993.
%%%%%%%%%%%%%%%%%%%%%%%%%%%%%%%%%%%%%%%%%%%%%%%%%%%%%%%%%%%%%%%%%%%%%%%
% Data for surge equation 
h.Xudot  	= -17400.0 ;
h.Xuau     	= -1.96e+003 ;
h.Xvr    	=  0.33 * mass ;
   
% Hydrodynamic coefficients in sway equation
h.Yvdot = -393000 ; 
h.Ypdot = -296000 ; 
h.Yrdot = -1400000 ; 
h.Yauv  = -11800 ; 
h.Yur   =  131000 ; 
h.Yvav  = -3700 ; 
h.Yrar   =  0 ;
h.Yvar  = -794000 ; 
h.Yrav  = -182000 ; 
h.Ybauv =  10800 ; % Y_{\phi |v u|}
h.Ybaur =  251000 ; 
h.Ybuu  = -74 ; 


% Hydrodynamic coefficients in yaw equation
h.Nvdot =  538000 ;
h.Npdot =  0 ;
h.Nrdot = -38.7e6;
h.Nauv  = -92000 ;
h.Naur  = -4710000 ;
h.Nvav  =  0 ;
h.Nrar  = -202000000 ;
h.Nvar  =  0 ;
h.Nrav  = -15600000 ;
h.Nbauv = -214000 ;
h.Nbuar = -4980000 ;
h.Nbuau = -8000 ;
%%%%%%%%%%%%%%%%%%%%%%%%%%%%%%%%%%%%%%%%%%%%%%%%%%%%%%%%%%%%%%%%%%%%%%%%%%%

au = abs(u);
av = abs(v); 
ar = abs(r);
b = 0;

% Hydrodynamic forces without added mass terms (considered in the M matrix)
Xh  = h.Xuau*u*au+h.Xvr*v*r;

Yh = h.Yauv*au*v + h.Yur*u*r + h.Yvav*v*av + h.Yvar*v*ar + h.Yrav*r*av ...
   + h.Ybauv*b*abs(u*v) + h.Ybaur*b*abs(u*r) + h.Ybuu*b*u^2;

Nh = h.Nauv*au*v + h.Naur*au*r + h.Nrar*r*ar + h.Nrav*r*av...
   +h.Nbauv*b*abs(u*b) + h.Nbuar*b*u*ar + h.Nbuau*b*u*au;

end

== matlab function Final_ShipModel_R19/Ship dynamics/Pod-Propellers/propL/Calculate Advance Ratio J/MATLAB Function2 ==
  data: n input; D input; ub input; J output
function J = fcn(n,D,ub)
    J =ub/(n*D) ;
end

== matlab function Final_ShipModel_R19/Ship dynamics/Pod-Propellers/propL/Projection T1 ==
  data: alpha input; T input; Fx output; Fy output
function [Fx, Fy] = fcn(alpha, T)

Fx = T*cos(alpha);

Fy = T*sin(alpha);

== matlab function Final_ShipModel_R19/Ship dynamics/Pod-Propellers/propL/Thrust/MATLAB Function ==
  data: RPM input; D input; K_T input; T output
function T = fcn(RPM, D, K_T)

RPS = RPM/60;

rho = 1020; % water density

T = K_T*rho*RPS^2*D^4;

== matlab function Final_ShipModel_R19/Ship dynamics/Pod-Propellers/propR/Calculate Advance Ratio J/MATLAB Function1 ==
  data: alpha input; u input; v input; ua output; r input; xp input; yp input
function ua = fcn(alpha, u, v ,r , xp , yp)
    
    uax = u + yp*r;     % Uax is velocity of propeller projected on x
    uay = v - xp*r;     % Uay is velocity of propeller projected on y
    phi = atan(uay/uax);    % Angle between ship velocity and x axis
    beta = phi - alpha;     % Angle difference between ship velocity and propeller's thrust

    ua = abs(hypot(uax,uay)*cos(beta)); % project ua on direction velocity of ship
end

== matlab function Final_ShipModel_R19/Autopilot/Autopilot/Integral trigger ==
  data: yaw input; trigger output; threshold input
function trigger = fcn(yaw, threshold)

if abs(yaw) < threshold
   trigger = 0;   % Trigger Integral part of PID
else
   trigger = 1;   % Stop Integral part of PID
end

end

== matlab function Final_ShipModel_R19/Ship dynamics/Pod-Propellers/propR/Calculate Advance Ratio J/MATLAB Function2 ==
  data: n input; D input; ub input; J output
function J = fcn(n,D,ub)
    J =ub/(n*D) ;
end

== matlab function Final_ShipModel_R19/Path tracking/Path following/Beta Calculation ==
  data: L input; beta output; shipPos input; SL output
function [beta, SL] = fcn(L, shipPos)

% N = shipPos' + [500 0]; % arbitrary point on the North axis of the ship
SL = L - shipPos'; % lookahead vector
% SN = N - shipPos'; % North vector
% SN = [500;0];
% beta = acos( dot(SN,SL) / (norm(SN)*norm(SL)) );
beta = atan2(SL(2), SL(1)); % angle between 2 vectors

% Determine correct sign for beta
% if L(1) < shipPos(1)
%    beta = -beta;
% end

== matlab function Final_ShipModel_R19/Path tracking/Path following/Line formula ==
  data: wayPoint1 input; line output; wayPoint2 input
function line = fcn(wayPoint1, wayPoint2)

% line = [0 0 0];

if (wayPoint2(1) == wayPoint1(1)) % Vertical line x - c = 0
   a = 1;
   b = 0;
else % Horizontal and diagonal line
   a = (wayPoint2(2) - wayPoint1(2)) / (wayPoint2(1) - wayPoint1(1));
   b = -1;
end

c = -(b*wayPoint1(2) + a*wayPoint1(1));

line = [a, b, c];
% ax + by + c = 0

== matlab function Final_ShipModel_R19/Ship dynamics/Pod-Propellers/propR/Thrust1/MATLAB Function ==
  data: RPM input; D input; K_T input; T output
function T = fcn(RPM, D, K_T)

RPS = RPM/60;

rho = 1020; % water density

T = K_T*rho*RPS^2*D^4;

== matlab function Final_ShipModel_R19/Ship dynamics/Pod-Propellers/propR/Projection T1 ==
  data: alpha input; T input; Fx output; Fy output
function [Fx, Fy] = fcn(alpha, T)

Fx = T*cos(alpha);

Fy = T*sin(alpha);

== matlab function Final_ShipModel_R19/Path tracking/Path following/Lookahead point ==
  data: wayPoint1 input; wayPoint2 input; L output; H input; l input
function L = fcn(wayPoint1, wayPoint2, H, l)
% L = [0 0]
AB = [(wayPoint2(1) - wayPoint1(1)), (wayPoint2(2) - wayPoint1(2))];
U = AB / norm(AB);
L = H + (5*l)*U;

== matlab function Final_ShipModel_R19/Path tracking/Path following/Projected point ==
  data: line input; H output; shipPos input
function H = fcn(line, shipPos) 

A = [line(1) line(2); line(2) -line(1)];
B = [-line(3); line(2)*shipPos(1) - line(1)*shipPos(2)];
H = transpose(A\B);

== matlab function Final_ShipModel_R19/Path tracking/Path following/MATLAB Function3 ==
  data: x output; u input; wp1 input; y output; line input
function [x, y] = fcn(u, wp1, line)
if (line(2) == 0)
   x = -line(3);
   y = u + wp1(2);
else
   x = u + wp1(1);
   y = line(1)*x + line(3);
end

== matlab function Final_ShipModel_R19/Ship dynamics/Supply vessel dynamics/MATLAB Function ==
  data: velo input; beta_estimated output
function beta_estimated = fcn(velo)

beta_estimated = atan2(velo(2), velo(1));

== matlab function Final_ShipModel_R19/Path tracking/Path following/MATLAB Function ==
  data: shipPos input; dis output; H input
function dis = fcn(shipPos, H)

dis = sqrt( (shipPos(1)-H(1))^2 + (shipPos(2)-H(2))^2);

== matlab function Final_ShipModel_R19/Observer/Sensor Model(Supply vessel2)/Coriolis/MATLAB Function ==
  data: u input; C1 output; C2 output; C3 output; v input; r input
function [C1,    C2,    C3]    = fcn(u,v,r)

% u = nu(1);
% v = nu(2);
% r = nu(3);

x_g = 0;
m = 357.0*1014;

C = [0                 0  -m*(x_g*r + v); ...
     0                 0             m*u; ...
     m*(x_g*r + v)  -m*u              0];

Co = C*[u;v;r];
C1 = Co(1);
C2 = Co(2);
C3 = Co(3);

end

% Xc =   h.m*(r*v+h.xG*r^2-h.zG*p*r);  
% Yc = - h.m*u*r;
% Kc =   h.m*h.zG*u*r;
% Nc = - h.m*h.xG*u*r;

== matlab function Final_ShipModel_R19/Path tracking/Path following/MATLAB Function1 ==
  settings: updateMethod=DISCRETE
  data: wayPoint2 input; H input; dist data_store_memory; dist1 output
function dist1 = fcn(wayPoint2, H)

% changePath = [0; 0]
global dist;
dist = sqrt((wayPoint2(1) - H(1))^2 + (wayPoint2(2) - H(2))^2);
dist1 = dist;
% changePath = 1;
% if dist < 250
%    changePath = [1, 0];
% end
% 
% changePath = [0 0]
% 
% if (dist < 250)
%    trig = 1;
% else
%    trig = 0;
% end

== matlab function Final_ShipModel_R19/Path tracking/Path assigning ==
  settings: updateMethod=DISCRETE
  data: path input; wp1 output; wp2 output; stop output; dist input
function [wp1, wp2, stop] = fcn(path, dist)
% global dist

wp1 = path(1,:)';
wp2 = path(2,:)';
stop = 0;

persistent current
if isempty(current)
   current = 0;
end
persistent change
if isempty(change)
   change = 1;
elseif dist < 250
%    disp(['dist < 250'])
   change = 1;
elseif dist > 250
   change = 0;
end

% change1 = change;
% current1 = current;

if change
%    disp('changed')
   current = current + 1
   if current == size(path,1)
%       current1
%       disp('exceed')
      stop = 1;
      return
   else
      wp1 = path(current,:)';
      wp2 = path(current+1,:)';
   end
else
%    disp('not change')
   wp1 = path(current,:)';
   wp2 = path(current+1,:)';
end


if dist > 250
%    disp(['dist > 250 '])
   change = 0;
end

% 
% change1 = change;
% current1 = current;
% y1 = [0;0];
% y2 = [0;0];
% persistent current
% persistent change
% if isempty(current)
%    current = 0
%    change = 1;
% end
% change
% persistent s
% s = size(wayPoints,1);
%
% if (dist < 250)
%    change = 1;
% end
%
% if change
%    current = current + 1
%    if current == s
%       stop = 1
%       disp('exceed')
%       return
%    else
%       wayPoint1 = wayPoints(current,:)'
%       wayPoint2 = wayPoints(current+1,:)'
%    end
% else
%    wayPoint1 = wayPoints(current,:)'
%    wayPoint2 = wayPoints(current+1,:)'
% end
%
% if (dist > 250)
%    change = 0;
% end

== matlab function Final_ShipModel_R19/Observer/Sensor Model(Supply vessel2)/HydEff/MATLAB Function ==
  data: mass input; Xh output; Yh output; Nh output; u input; v input; r input
function [Xh, Yh, Nh] = fcn(mass, u, v, r)

%%%%%%%%%%%%%%%%%%%%%%%%%%%%%%%%%%%%%%%%%%%%%%%%%%%%%%%%%%%%%%%%%%%%%%%
% The hydrodynamic derivatives are given in dimensional form, and follow
% from the original publication of Blanke and Christensen 1993.
%%%%%%%%%%%%%%%%%%%%%%%%%%%%%%%%%%%%%%%%%%%%%%%%%%%%%%%%%%%%%%%%%%%%%%%
% Data for surge equation 
h.Xudot  	= -17400.0 ;
h.Xuau     	= -1.96e+003 ;
h.Xvr    	=  0.33 * mass ;
   
% Hydrodynamic coefficients in sway equation
h.Yvdot = -393000 ; 
h.Ypdot = -296000 ; 
h.Yrdot = -1400000 ; 
h.Yauv  = -11800 ; 
h.Yur   =  131000 ; 
h.Yvav  = -3700 ; 
h.Yrar   =  0 ;
h.Yvar  = -794000 ; 
h.Yrav  = -182000 ; 
h.Ybauv =  10800 ; % Y_{\phi |v u|}
h.Ybaur =  251000 ; 
h.Ybuu  = -74 ; 


% Hydrodynamic coefficients in yaw equation
h.Nvdot =  538000 ;
h.Npdot =  0 ;
h.Nrdot = -38.7e6;
h.Nauv  = -92000 ;
h.Naur  = -4710000 ;
h.Nvav  =  0 ;
h.Nrar  = -202000000 ;
h.Nvar  =  0 ;
h.Nrav  = -15600000 ;
h.Nbauv = -214000 ;
h.Nbuar = -4980000 ;
h.Nbuau = -8000 ;
%%%%%%%%%%%%%%%%%%%%%%%%%%%%%%%%%%%%%%%%%%%%%%%%%%%%%%%%%%%%%%%%%%%%%%%%%%%

au = abs(u);
av = abs(v); 
ar = abs(r);
b = 0;

% Hydrodynamic forces without added mass terms (considered in the M matrix)
Xh  = h.Xuau*u*au+h.Xvr*v*r;

Yh = h.Yauv*au*v + h.Yur*u*r + h.Yvav*v*av + h.Yvar*v*ar + h.Yrav*r*av ...
   + h.Ybauv*b*abs(u*v) + h.Ybaur*b*abs(u*r) + h.Ybuu*b*u^2;

Nh = h.Nauv*au*v + h.Naur*au*r + h.Nrar*r*ar + h.Nrav*r*av...
   +h.Nbauv*b*abs(u*b) + h.Nbuar*b*u*ar + h.Nbuau*b*u*au;

end

== matlab function Final_ShipModel_R19/Observer/Sensor Model(Supply vessel2)/M_inv/MATLAB Function ==
  data: Minv output; mass input; Izz input
function Minv = fcn(mass, Izz)

h.m   = mass;    % Mass [Kg]
h.Izz = Izz;     % Yaw Inertia
h.xG  = 0;

%%%%%%%%%%%%%%%%%%%%%%%%%%%%%%%%%%%%%%%%%%%%%%%%%%%%%%%%%%%%%%%%%%%%%%%
% The hydrodynamic derivatives are given in dimensional form, and follow
% from the original publication of Blanke and Christensen 1993.
%%%%%%%%%%%%%%%%%%%%%%%%%%%%%%%%%%%%%%%%%%%%%%%%%%%%%%%%%%%%%%%%%%%%%%%
% Data for surge equation 
h.Xudot  	= -17400.0;
% h.Xuau     	= -1.96e+003;
% h.Xvr    	=  0.33 * mass;
   
% Hydrodynamic coefficients in sway equation
h.Yvdot = -393000; 
h.Ypdot = -296000; 
h.Yrdot = -1400000; 
% h.Yauv  = -11800; 
% h.Yur   =  131000; 
% h.Yvav  = -3700; 
% h.Yrar  =  0;
% h.Yvar  = -794000; 
% h.Yrav  = -182000; 
% h.Ybauv =  10800; % Y_{\phi |v u|}
% h.Ybaur =  251000; 
% h.Ybuu  = -74;


% Hydrodynamic coefficients in yaw equation
h.Nvdot =  538000;
h.Npdot =  0;
h.Nrdot = -38.7e6;
% h.Nauv  = -92000;
% h.Naur  = -4710000;
% h.Nvav  =  0;
% h.Nrar  = -202000000;
% h.Nvar  =  0;
% h.Nrav  = -15600000;
% h.Nbauv = -214000;
% h.Nbuar = -4980000;
% h.Nbuau = -8000;
%%%%%%%%%%%%%%%%%%%%%%%%%%%%%%%%%%%%%%%%%%%%%%%%%%%%%%%%%%%%%%%%%%%%%%%%%%%


M = [(h.m-h.Xudot)                  0                  0; ...
                 0      (h.m-h.Yvdot) (h.m*h.xG-h.Yrdot); ...
                 0 (h.m*h.xG-h.Nvdot)    (h.Izz-h.Nrdot)];

Minv = inv(M);
end
